simulink model "revo_driver_test"  (Simulink 7.5)
settings: Solver=FixedStepDiscrete  SolverMode=SingleTasking  StartTime=0.0  StopTime=10.0  FixedStep=0.01  RelTol=1e-3
undefined symbols (not defined in the file): getRevoData, Init_onlyOnce, Init_Reset, initUart1ForRevo, processNewRevoData, y1
libraries: dsPICdrivers x7, simulink x1
CloseFcn:
  | rtwprivate ssgencode ModelCloseRequest code_gen
settings Model: Creator=bwmairs  LastModifiedBy=Bryant  BufferReuse=off
settings OptimizationCC: InlineParams=on  InlineInvariantSignals=on  OptimizeBlockIOStorage=off  BufferReuse=off  ExpressionFolding=off  LocalBlockOutputs=off  ZeroExternalMemoryAtStartup=off  ZeroInternalMemoryAtStartup=off  NoFixptDivByZeroProtection=on  EfficientFloat2IntCast=on  OptimizeModelRefInitCode=on
settings DebuggingCC: ReadBeforeWriteMsg=DisableAll  WriteAfterWriteMsg=DisableAll  WriteAfterReadMsg=DisableAll  ParameterOverflowMsg=warning  UniqueDataStoreMsg=error
settings HardwareCC: ProdBitPerInt=16  ProdIntDivRoundTo=Zero  ProdEndianess=LittleEndian  ProdWordSize=16  ProdHWDeviceType=16-bit Generic
settings RTWCC: SystemTargetFile=dspic.tlc  MakeCommand=make_CreateMPLAB  TemplateMakefile=dspic_pic30_gcc.tmf  PostCodeGenCommand=dsPIC_Compile()  Description=Embedded Target for Microchip dsPIC (real-time)  ProcessScript=dspic_make_rtw_hook  RTWCompilerOptimization=On
settings RTWCC: CustomSource=|
  | ../../../../../ECAN_dspic/circBuffer.c
  | ../../clib/conversions.c
  | ../../clib/nmea.c
  | ../../clib/revo.c
  | ../../clib/uart1.c
settings CodeAppCC: IgnoreCustomStorageClasses=off  IgnoreTestpoints=on
settings STFCustomTargetCC: TargetFunctionLibrary=C89/C90 (ANSI)  IncludeMdlTerminateFcn=off  CombineOutputUpdateFcns=on  SuppressErrorStatus=on  ERTCustomFileBanners=on  SupportAbsoluteTime=off  SupportNonFinite=off  SupportComplex=off  SupportContinuousTime=off  SupportNonInlinedSFcns=off  SystemTargetFile=dspic.tlc
settings ERTTargetCC: TargetFunctionLibrary=C89/C90 (ANSI)  MultiwordLength=2048  ParMdlRefBuildCompliant=off  CompOptLevelCompliant=off  IncludeMdlTerminateFcn=off  SuppressErrorStatus=on  ERTFirstTimeCompliant=off  SupportAbsoluteTime=off  SupportNonFinite=off  SupportComplex=off  ModelStepFunctionPrototypeControlCompliant=off  CPPClassGenCompliant=off  ExtModeMexFile=ext_serial_win32_comm  InlinedParameterPlacement=NonHierarchical  ERTSrcFileBannerTemplate=dsPIC_code_template.cgt  ERTHdrFileBannerTemplate=dsPIC_code_template.cgt  ERTDataSrcFileTemplate=dsPIC_code_template.cgt  ERTDataHdrFileTemplate=dsPIC_code_template.cgt  ERTCustomFileTemplate=dsPIC_main.tlc
settings CustomProperty: DataType=string  Value=C:\PROGRA~1\MATLAB\R2010a\bin\win64\gmake

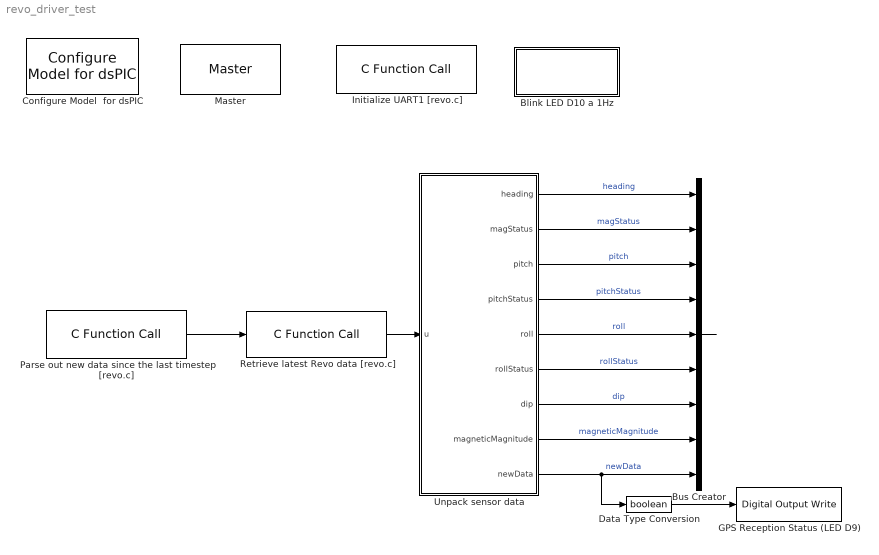
== system revo_driver_test ==
  Blink LED D10 a 1Hz : Subsystem
      mask Display: disp('blink');
  Bus Creator : BusCreator  Inputs=9
  Configure Model  for dsPIC : dsPICdrivers/Simulink Configuration/Configure Model  for dsPIC
  Data Type Conversion : DataTypeConversion  OutDataTypeMode=boolean  OutDataType=fixdt(1, 16)  OutScaling=2^0  OutDataTypeStr=boolean  RndMeth=Simplest
  GPS Reception Status (LED D9) : dsPICdrivers/Digital I//O/Digital Output Write  Tag=dsPIC_Digital_Output  Priority=5  PORT=A  Pin=[6]  Simultaneous=off  OrderingInOutPopup=None
  Initialize UART1 [revo.c] : dsPICdrivers/OTHERS/C Function Call  Tag=dsPIC_dsPIC_CFunctionCall  FctUpdate=None  fctName=processNewRevoData  INPUT_SIZE=1  INPUT1=--  INPUT2=--  INPUT3=--  OUTPUT_SIZE=1  OUTPUT1=--  SampleTime=0.01  InputType=[]  OutputType=[]  FctDeclaration=extern void processNewRevoData();  FctCall=processNewRevoData();  OrderingInOutPopup=None  FctStart=Start Function (Call once and only once)  FctStart_Name=initUart1ForRevo  FctStart_Declaration=inline extern void initUart1ForRevo();  FctStart_Call=initUart1ForRevo();  FctInit=None  FctInit_Name=Init_Reset  FctInit_Declaration=inline extern void Init_Reset();  FctInit_Call=Init_Reset();  PinDigitalInput=[]  PinDigitalOutput=[]  AnalogueInput=[]
  Master : dsPICdrivers/Master  Tag=dsPIC_MASTER  Priority=1  TimeStepType=Timer1  picType=33fJ256GP710A  fcy=40000000  Quartz_33f=8e6  PLLActive_33f=on  fcyDesired_33f=40000000  tmr1="[8  49999  0]"  tmr1Info="Time Step : 0.01  ;   Error : 0%  PR1=49999"  tmr2345="[0  0  0  0  0  0  0  0]"  tmr2345cfg=[-1 -1 -1 -1 -1 -1 -1 -1]  IOautoConf=on  typePort="[ 0   0   0   0   0   0  10  10   0   0   0   0   0   0   0   0   0   0   0   0   0   0   0   0   0   0   0   0   0   0   0   0   0   0   0   0   0   0   0   0   0   0   0   0   0   0   0   0   0   0   0   0   0   0   0   0   0   0   0   0   0   0   0   0   0   0   0   0   0   0   0   0   0   0   0   0   0   0   0   0   0   0   0   0   0   0   0   0   0   0   0   0   0   0   0   0   0   0   0   0   0   0   0   0   0   0   0   0   0   0   0   0 ]"  TRIS="[ 65343  65535  65535  65535  65535  65535  65535 ]"  ADPCFG=12582912  MasterBusyPort=None  MasterOverloadPort=None  FOSC=Quartz (XT - HS)  ClockSwitchMonitor=Both disabled  TempProtection_33f=TEMP_ON  FPBOR=<empty>  PWRT=disable  MCLR=<empty>  ICD=ICS_PGD1  JTAGEN=JTAGEN_OFF  PowerSave=off  OverrideFcy=off  NewFcy=1e6  PR2345="[65535  65535  65535  65535  65535  65535  65535  65535]"
  Parse out new data since the last timestep [revo.c] : dsPICdrivers/OTHERS/C Function Call  Tag=dsPIC_dsPIC_CFunctionCall  FctUpdate=Output Function  fctName=processNewRevoData  INPUT_SIZE=1  INPUT1=--  INPUT2=--  INPUT3=--  OUTPUT_SIZE=1  OUTPUT1=--  SampleTime=0.01  InputType=[ ]  OutputType=[ ]  FctDeclaration=extern void processNewRevoData();  FctCall=processNewRevoData();  OrderingInOutPopup=Output  FctStart=None  FctStart_Name=Init_onlyOnce  FctStart_Declaration=inline extern void Init_onlyOnce();  FctStart_Call=Init_onlyOnce();  FctInit=None  FctInit_Name=Init_Reset  FctInit_Declaration=inline extern void Init_Reset();  FctInit_Call=Init_Reset();  PinDigitalInput=[]  PinDigitalOutput=[]  AnalogueInput=[]
  Retrieve latest Revo data [revo.c] : dsPICdrivers/OTHERS/C Function Call  Tag=dsPIC_dsPIC_CFunctionCall  FctUpdate=Output Function  fctName=getRevoData  INPUT_SIZE=1  INPUT1=--  INPUT2=--  INPUT3=--  OUTPUT_SIZE=22  OUTPUT1=uint8  SampleTime=0.01  InputType=[ ]  OutputType=[ 2 ]  FctDeclaration=extern void getRevoData(uint8_T* y1);  FctCall=getRevoData(*%y1);  OrderingInOutPopup=Input  FctStart=None  FctStart_Name=Init_onlyOnce  FctStart_Declaration=inline extern void Init_onlyOnce();  FctStart_Call=Init_onlyOnce();  FctInit=None  FctInit_Name=Init_Reset  FctInit_Declaration=inline extern void Init_Reset();  FctInit_Call=Init_Reset();  PinDigitalInput=[]  PinDigitalOutput=[]  AnalogueInput=[]
  Unpack sensor data : Stateflow chart  TreatAsAtomicUnit=on
  wires:
  Bus Creator/1 -> ?
  Parse out new data since the last timestep [revo.c]/1 -> Retrieve latest Revo data [revo.c]/1
  Data Type Conversion/1 -> GPS Reception Status (LED D9)/1
  Unpack sensor data/4(pitchStatus) -> Bus Creator/4  "pitchStatus"
  Unpack sensor data/5(roll) -> Bus Creator/5  "roll"
  Unpack sensor data/6(rollStatus) -> Bus Creator/6  "rollStatus"
  Unpack sensor data/7(dip) -> Bus Creator/7  "dip"
  Unpack sensor data/8(magneticMagnitude) -> Bus Creator/8  "magneticMagnitude"
  Unpack sensor data/9(newData) -> Bus Creator/9, Data Type Conversion/1  "newData"
  Retrieve latest Revo data [revo.c]/1 -> Unpack sensor data/1(u)
  Unpack sensor data/1(heading) -> Bus Creator/1  "heading"
  Unpack sensor data/2(magStatus) -> Bus Creator/2  "magStatus"
  Unpack sensor data/3(pitch) -> Bus Creator/3  "pitch"

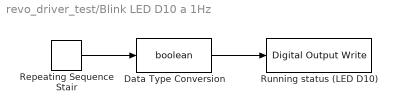
== system revo_driver_test/Blink LED D10 a 1Hz ==
  Data Type Conversion : DataTypeConversion  OutDataTypeMode=boolean  OutDataType=sfix(16)  OutScaling=2^0  OutDataTypeStr=boolean  RndMeth=Simplest
  Repeating Sequence Stair : simulink/Sources/Repeating Sequence Stair  SystemSampleTime=-1  OutValues=[1 0]  tsamp=1  OutMin=[]  OutMax=[]  OutDataTypeStr=double  OutputDataTypeScalingMode=double  OutDataType=fixdt(0,8)  ConRadixGroup=Best Precision: Vector-wise  OutScaling=2^-12
  Running status (LED D10) : dsPICdrivers/Digital I//O/Digital Output Write  Tag=dsPIC_Digital_Output  Priority=5  PORT=A  Pin=[7]  Simultaneous=off  OrderingInOutPopup=None
  wires:
  Repeating Sequence Stair/1 -> Data Type Conversion/1
  Data Type Conversion/1 -> Running status (LED D10)/1

== matlab function Unpack sensor data ==
  data: heading output double; magStatus output double; pitch output double; pitchStatus output double; roll output double; rollStatus output double; dip output double; magneticMagnitude output double; newData output double; u input uint8
function [heading, magStatus, pitch, pitchStatus, roll, rollStatus, dip, magneticMagnitude, newData] = unpack(u)
%#eml

heading = typecast(u(1:4), 'single');
magStatus = u(5);
pitch = typecast(u(6:9), 'single');
pitchStatus = u(10);
roll = typecast(u(11:14), 'single');
rollStatus = u(15);
dip = typecast(u(16:19), 'single');
magneticMagnitude = typecast(u(20:21), 'uint16');
newData = u(22);
